simulink model "simulacion"  (R2018a)
settings: Solver=VariableStepAuto  StartTime=0.0  StopTime=10.0  RelTol=1e-3
undefined symbols (not defined in the file): motor, planta_y, planta_ysp
settings Model: Creator=seba  LastModifiedBy=seba

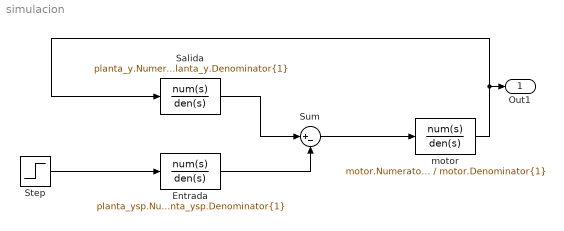
== system simulacion ==
  Entrada : TransferFcn  Numerator=planta_ysp.Numerator{1}  Denominator=planta_ysp.Denominator{1}  ContinuousStateAttributes=Entrada
  Salida : TransferFcn  Numerator=planta_y.Numerator{1}  Denominator=planta_y.Denominator{1}  ContinuousStateAttributes=salida
  Step : Step  SampleTime=0
  Sum : Sum  Inputs=|+-
  motor : TransferFcn  Numerator=motor.Numerator{1}  Denominator=motor.Denominator{1}  ContinuousStateAttributes=motor
  Out1 : Outport  SignalName=sistema_salida
  wires:
  Salida/1 -> Sum/1
  Entrada/1 -> Sum/2
  Sum/1 -> motor/1
  motor/1 -> Out1/1, Salida/1
  Step/1 -> Entrada/1
